simulink model "AM_Radio_Receiver"  (R2024b)
settings: Solver=VariableStepAuto  StartTime=0.0  StopTime=10.0  RelTol=1e-3
settings Model: Creator=memdus  LastModifiedBy=memdus

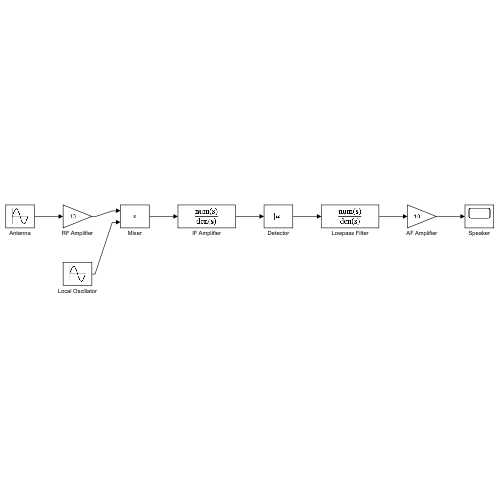
[thumbnail: Simulink's stored preview of the top-level diagram]
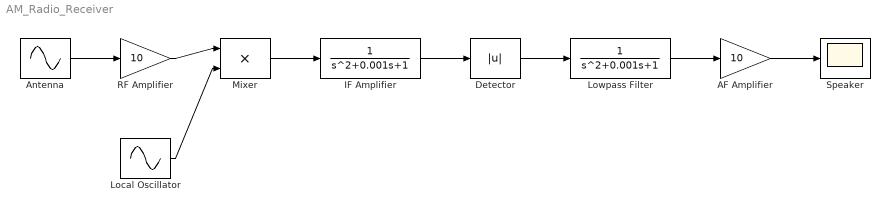
== system AM_Radio_Receiver ==
  AF Amplifier : Gain  Gain=10
  Antenna : Sin  SampleTime=0
  Detector : Abs  SaturateOnIntegerOverflow=off
  IF Amplifier : TransferFcn  Numerator=1  Denominator=[1 0.001 1]
  Local Oscillator : Sin  SampleTime=0
  Lowpass Filter : TransferFcn  Numerator=1  Denominator=[1 0.001 1]
  Mixer : Product
  RF Amplifier : Gain  Gain=10
  Speaker : Scope
  wires:
  Antenna/1 -> RF Amplifier/1
  RF Amplifier/1 -> Mixer/1
  Local Oscillator/1 -> Mixer/2
  Mixer/1 -> IF Amplifier/1
  IF Amplifier/1 -> Detector/1
  Detector/1 -> Lowpass Filter/1
  Lowpass Filter/1 -> AF Amplifier/1
  AF Amplifier/1 -> Speaker/1
